simulink model "chap5_1sim"  (R2016b)
settings: Solver=FixedStepAuto  StartTime=0.0  StopTime=RunTime  FixedStep=0.01  MaxStep=0.05  RelTol=1e-3  EnableMultiTasking=on
settings Model: Creator=Masoud  LastModifiedBy=Hafez
settings DataIOCC: LimitDataPoints=on  SaveFormat=Array
settings OptimizationCC: LifeSpan=inf
settings DebuggingCC: InheritedTsInSrcMsg=none  SFUnexpectedBacktrackingDiag=warning  SFNoUnconditionalDefaultTransitionDiag=warning  SFExecutionAtInitializationDiag=none
settings HardwareCC: ProdBitPerPointer=32  ProdBitPerSizeT=32  ProdBitPerPtrDiffT=32  ProdLargestAtomicFloat=None  ProdIntDivRoundTo=Undefined  ProdEndianess=Unspecified  ProdWordSize=32  ProdHWDeviceType=32-bit Generic
settings ModelReferenceCC: PropagateSignalLabelsOutOfModel=off
settings GRTTargetCC: TargetLangStandard=C89/C90 (ANSI)  GeneratePreprocessorConditionals=Disable all
settings ConfigComp: CovMetricSettings=dw  CovHtmlReporting=on  CovSaveCumulativeToWorkspaceVar=on  CovSaveSingleToWorkspaceVar=on  CovExternalEMLEnable=off

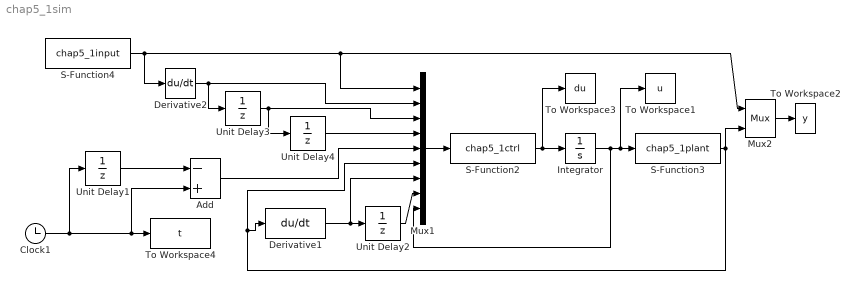
== system chap5_1sim ==
  Add : Sum  Inputs=-+
  Clock1 : Clock
  Derivative1 : Derivative
  Derivative2 : Derivative
  Integrator : Integrator
  Mux1 : Mux  Inputs=9
  Mux2 : Mux  Inputs=2
  S-Function2 : S-Function  FunctionName=chap5_1ctrl  SFunctionModules='chap5_1ctrl'  SFunctionDeploymentMode=off  EnableBusSupport=off
  S-Function3 : S-Function  FunctionName=chap5_1plant  SFunctionModules='chap5_1plant'  SFunctionDeploymentMode=off  EnableBusSupport=off
  S-Function4 : S-Function  FunctionName=chap5_1input  SFunctionModules='chap5_1nput'  SFunctionDeploymentMode=off  EnableBusSupport=off
  To Workspace1 : ToWorkspace  VariableName=u  SampleTime=-1
  To Workspace2 : ToWorkspace  VariableName=y  SampleTime=-1
  To Workspace3 : ToWorkspace  VariableName=du  SampleTime=-1
  To Workspace4 : ToWorkspace  VariableName=t  SampleTime=-1
  Unit Delay{1..4} (4 alike) : UnitDelay  SampleTime=-1
  wires:
  Mux1/1 -> S-Function2/1
  Mux2/1 -> To Workspace2/1
  Unit Delay2/1 -> Mux1/8
  Derivative1/1 -> Mux1/7, Unit Delay2/1
  S-Function3/1 -> Derivative1/1, Mux1/6, Mux2/2
  Integrator/1 -> S-Function3/1, To Workspace1/1, Mux1/9
  S-Function4/1 -> Derivative2/1, Mux1/1, Mux2/1
  Derivative2/1 -> Mux1/2, Unit Delay3/1
  Unit Delay3/1 -> Unit Delay4/1, Mux1/3
  Clock1/1 -> Unit Delay1/1, Add/2, To Workspace4/1
  Unit Delay1/1 -> Add/1
  Add/1 -> Mux1/5
  Unit Delay4/1 -> Mux1/4
  S-Function2/1 -> Integrator/1, To Workspace3/1
